simulink model "simulink_real_Estados_digital"  (R2023a)
settings: Solver=VariableStepAuto  StartTime=0.0  StopTime=10  RelTol=1e-3
undefined symbols (not defined in the file): A, B, C, D, K0d, Kd, TS
libraries: simulink x1
settings Model: Creator=Agustin  LastModifiedBy=Agustin

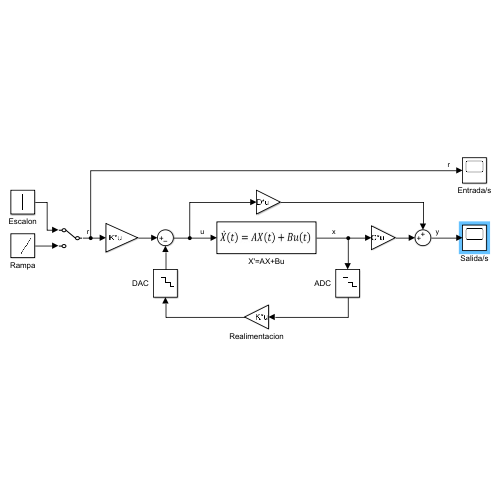
[thumbnail: Simulink's stored preview of the top-level diagram]
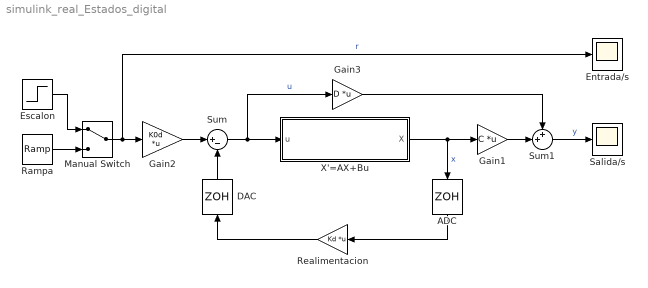
== system simulink_real_Estados_digital ==
  ADC : ZeroOrderHold  SampleTime=TS
  DAC : ZeroOrderHold  SampleTime=TS
  Entrada/s : Scope
  Escalon : Step  SampleTime=0
  Gain1 : Gain  Gain=C  Multiplication=Matrix(K*u)
  Gain2 : Gain  Gain=K0d  Multiplication=Matrix(K*u)
  Gain3 : Gain  Gain=D  Multiplication=Matrix(K*u)
  Manual Switch : ManualSwitch
  Rampa : simulink/Sources/Ramp  slope=1  start=0  InitialOutput=0
  Realimentacion : Gain  Gain=Kd  Multiplication=Matrix(K*u)
  Salida/s : Scope
  Sum : Sum  Inputs=|+-
  Sum1 : Sum  Inputs=++|
  X'=AX+Bu : Subsystem
      mask Display: image('$imagefile'); % Use "Edit Image" on toolstrip to change.
  wires:
  Escalon/1 -> Manual Switch/1
  Sum/1 -> X'=AX+Bu/1(u), Gain3/1  "u"
  Rampa/1 -> Manual Switch/2
  Manual Switch/1 -> Gain2/1, Entrada/s/1  "r"
  Gain2/1 -> Sum/1
  Realimentacion/1 -> DAC/1
  Sum1/1 -> Salida/s/1  "y"
  X'=AX+Bu/1(X) -> ADC/1, Gain1/1  "x"
  Gain1/1 -> Sum1/2
  Gain3/1 -> Sum1/1
  DAC/1 -> Sum/2
  ADC/1 -> Realimentacion/1

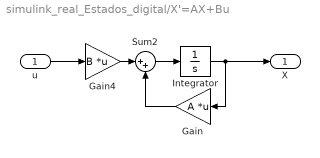
== system simulink_real_Estados_digital/X'=AX+Bu ==
  u : Inport
  Gain : Gain  Gain=A  Multiplication=Matrix(K*u)
  Gain4 : Gain  Gain=B  Multiplication=Matrix(K*u)
  Integrator : Integrator
  Sum2 : Sum  Inputs=|++
  X : Outport
  wires:
  Gain4/1 -> Sum2/1
  Integrator/1 -> X/1, Gain/1
  Sum2/1 -> Integrator/1
  Gain/1 -> Sum2/2
  u/1 -> Gain4/1
